simulink model "cmd_model"  (R2015a)
settings: configuration reference "config_cosim" (kept outside this file)
libraries: Sys_CMD x1
settings Model: Creator=ericli  LastModifiedBy=ericli
settings ConfigSetRef: SourceLocation=Base Workspace

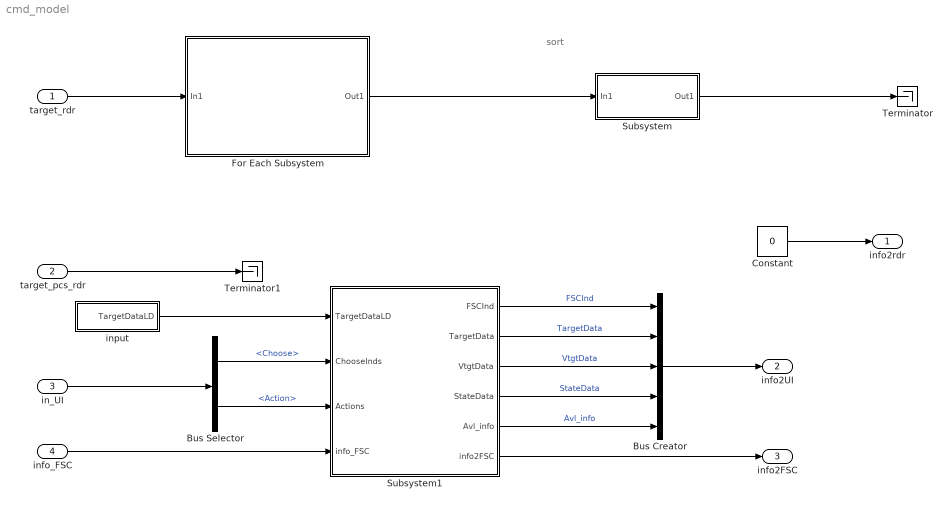
== system cmd_model ==
  note: sort
  target_rdr : Inport  OutDataTypeStr=Bus: BusObject_tgt_rdr2CC  PortDimensions=48  BusOutputAsStruct=on
  target_pcs_rdr : Inport  Port=2  OutDataTypeStr=Bus: BusObject_msg_pcs_rdr2CC  BusOutputAsStruct=on
  in_UI : Inport  Port=3  OutDataTypeStr=Bus: BusObject_input_UI  BusOutputAsStruct=on
  info_FSC : Inport  Port=4  OutDataTypeStr=Bus: BusObject_info_FSC2CC
  Bus Creator : BusCreator  Inputs=5  OutDataTypeStr=Bus: BusObject_info_CC2UI
      settings: InheritFromInputs=off
  Bus Selector : BusSelector  OutputSignals=Choose,Action
  Constant : Constant  Value=0  OutDataTypeStr=Bus:BusObject_info_CC2rdr  LockScale=on
  For Each Subsystem : Subsystem  TreatAsAtomicUnit=on
  Subsystem : Subsystem
  Subsystem1 : Subsystem
  Terminator : Terminator
  Terminator1 : Terminator
  input : Subsystem
  info2rdr : Outport  OutDataTypeStr=Bus: BusObject_info_CC2rdr  BusOutputAsStruct=on
  info2UI : Outport  Port=2  OutDataTypeStr=Bus: BusObject_info_CC2UI
  info2FSC : Outport  Port=3  OutDataTypeStr=Bus: BusObject_info_CC2FSC
  wires:
  target_rdr/1 -> For Each Subsystem/1(In1)
  For Each Subsystem/1(Out1) -> Subsystem/1(In1)
  Subsystem/1(Out1) -> Terminator/1
  Bus Creator/1 -> info2UI/1
  in_UI/1 -> Bus Selector/1
  Bus Selector/1 -> Subsystem1/2(ChooseInds)  "<Choose>"
  Bus Selector/2 -> Subsystem1/3(Actions)  "<Action>"
  info_FSC/1 -> Subsystem1/4(info_FSC)
  Subsystem1/6(info2FSC) -> info2FSC/1
  Constant/1 -> info2rdr/1
  Subsystem1/5(Avl_info) -> Bus Creator/5  "Avl_info"
  Subsystem1/4(StateData) -> Bus Creator/4  "StateData"
  Subsystem1/2(TargetData) -> Bus Creator/2  "TargetData"
  Subsystem1/1(FSCInd) -> Bus Creator/1  "FSCInd"
  input/1(TargetDataLD) -> Subsystem1/1(TargetDataLD)
  target_pcs_rdr/1 -> Terminator1/1
  Subsystem1/3(VtgtData) -> Bus Creator/3  "VtgtData"

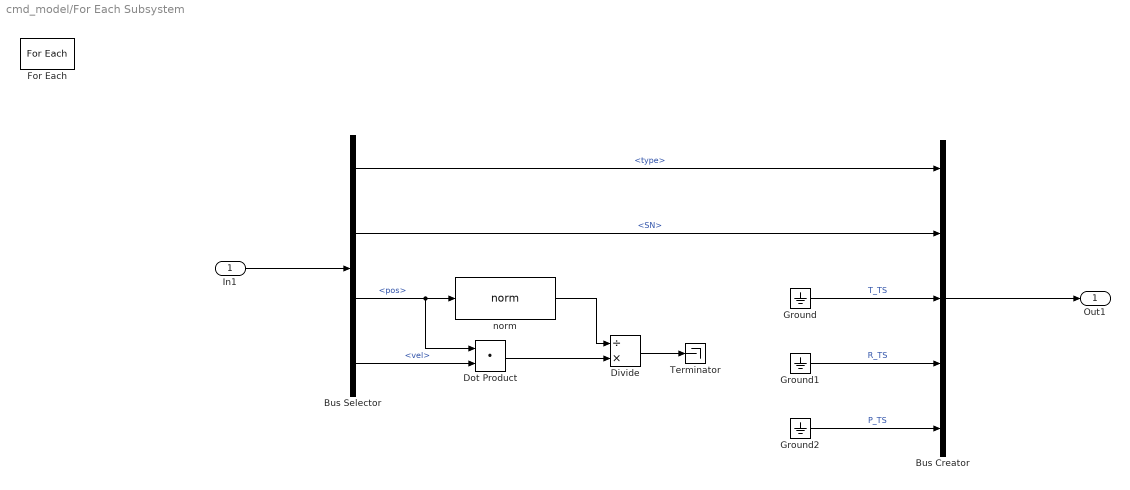
== system cmd_model/For Each Subsystem ==
  In1 : Inport  Partition=on  PartitionDimension=1  PartitionWidth=1
  Bus Creator : BusCreator  Inputs=5  OutDataTypeStr=Bus: bus_cmp_tgt  NonVirtualBus=on
      settings: InheritFromInputs=off
  Bus Selector : BusSelector  OutputSignals=type,SN,pos,vel
  Divide : Product  Inputs=/*
  Dot Product : DotProduct  InputSameDT=on  OutDataTypeStr=Inherit: Inherit via internal rule
  For Each : ForEach  DisableCoverage=on  IndexMode=One-based
  Ground : Ground
  Ground1 : Ground
  Ground2 : Ground
  Terminator : Terminator
  norm : Sys_CMD/norm
  Out1 : Outport  OutDataTypeStr=Bus: bus_cmp_tgt  ConcatenationDimension=1
  wires:
  In1/1 -> Bus Selector/1
  Bus Selector/3 -> norm/1, Dot Product/1  "<pos>"
  Bus Selector/4 -> Dot Product/2  "<vel>"
  norm/1 -> Divide/1
  Dot Product/1 -> Divide/2
  Divide/1 -> Terminator/1
  Bus Creator/1 -> Out1/1
  Bus Selector/1 -> Bus Creator/1  "<type>"
  Bus Selector/2 -> Bus Creator/2  "<SN>"
  Ground/1 -> Bus Creator/3  "T_TS"
  Ground1/1 -> Bus Creator/4  "R_TS"
  Ground2/1 -> Bus Creator/5  "P_TS"

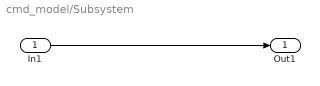
== system cmd_model/Subsystem ==
  In1 : Inport
  Out1 : Outport
  wires:
  In1/1 -> Out1/1

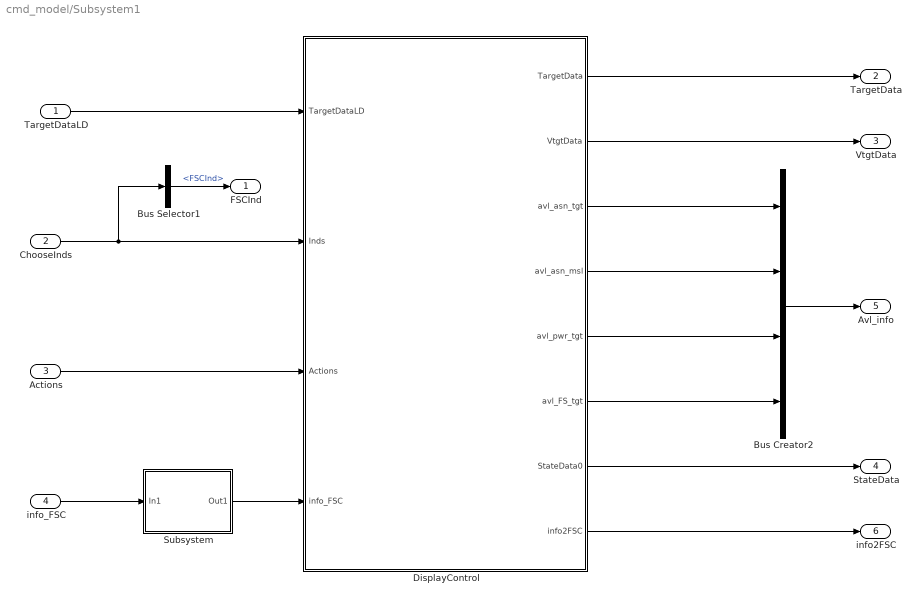
== system cmd_model/Subsystem1 ==
  TargetDataLD : Inport
  ChooseInds : Inport  Port=2  OutDataTypeStr=Bus:ChooseBusObject
  Actions : Inport  Port=3  OutDataTypeStr=Bus: ActionBusObject
  info_FSC : Inport  Port=4  OutDataTypeStr=Bus:BusObject_info_FSC2CC
  Bus Creator2 : BusCreator  OutDataTypeStr=Bus:AvlBusObject
  Bus Selector1 : BusSelector  OutputSignals=FSCInd
  DisplayControl : Stateflow chart  TreatAsAtomicUnit=on
  Subsystem : Subsystem
  FSCInd : Outport
  TargetData : Outport  Port=2
  VtgtData : Outport  Port=3
  StateData : Outport  Port=4  OutDataTypeStr=Bus:StateBusObject
  Avl_info : Outport  Port=5  OutDataTypeStr=Bus:AvlBusObject
  info2FSC : Outport  Port=6  OutDataTypeStr=Bus: BusObject_info_CC2FSC
  wires:
  DisplayControl/3(avl_asn_tgt) -> Bus Creator2/1
  DisplayControl/8(info2FSC) -> info2FSC/1
  DisplayControl/1(TargetData) -> TargetData/1
  Bus Creator2/1 -> Avl_info/1
  TargetDataLD/1 -> DisplayControl/1(TargetDataLD)
  DisplayControl/5(avl_pwr_tgt) -> Bus Creator2/3
  DisplayControl/7(StateData0) -> StateData/1
  DisplayControl/4(avl_asn_msl) -> Bus Creator2/2
  Bus Selector1/1 -> FSCInd/1  "<FSCInd>"
  ChooseInds/1 -> DisplayControl/2(Inds), Bus Selector1/1
  DisplayControl/6(avl_FS_tgt) -> Bus Creator2/4
  Actions/1 -> DisplayControl/3(Actions)
  DisplayControl/2(VtgtData) -> VtgtData/1
  info_FSC/1 -> Subsystem/1(In1)
  Subsystem/1(Out1) -> DisplayControl/4(info_FSC)

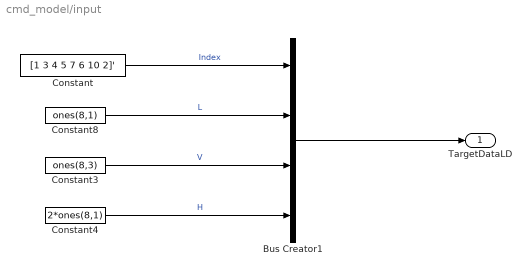
== system cmd_model/input ==
  Bus Creator1 : BusCreator  OutDataTypeStr=Bus: TgtDataLDBusObject  NonVirtualBus=on
  Constant : Constant  Value=[1 3 4 5 7 6 10 2]'  OutDataTypeStr=double
  Constant3 : Constant  Value=ones(8,3)  OutDataTypeStr=double
  Constant4 : Constant  Value=2*ones(8,1)  OutDataTypeStr=double
  Constant8 : Constant  Value=ones(8,1)  OutDataTypeStr=double
  TargetDataLD : Outport  OutDataTypeStr=Bus: TgtDataLDBusObject
  wires:
  Constant8/1 -> Bus Creator1/2  "L"
  Constant4/1 -> Bus Creator1/4  "H"
  Constant/1 -> Bus Creator1/1  "Index"
  Constant3/1 -> Bus Creator1/3  "V"
  Bus Creator1/1 -> TargetDataLD/1

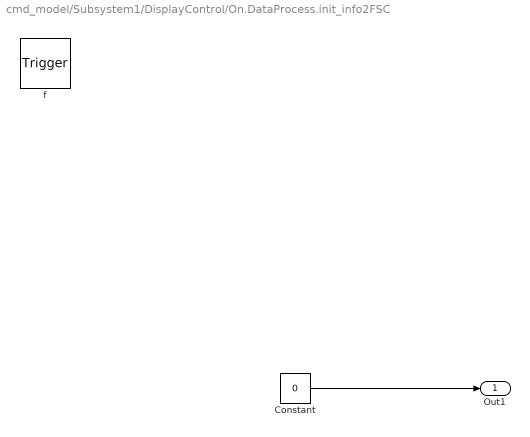
== system cmd_model/Subsystem1/DisplayControl/On.DataProcess.init_info2FSC ==
  f : TriggerPort  TriggerType=function-call
      settings: CopyFcn=Stateflow.SLINSF.SimulinkMan.removeBlockPreDeleteFcn  PreDeleteFcn=Stateflow.SLINSF.SimulinkMan.unsafePredeleteFcn
  Constant : Constant  Value=0  OutDataTypeStr=Bus: BusObject_info_CC2FSC
  Out1 : Outport  OutDataTypeStr=Bus: BusObject_info_CC2FSC
  wires:
  Constant/1 -> Out1/1

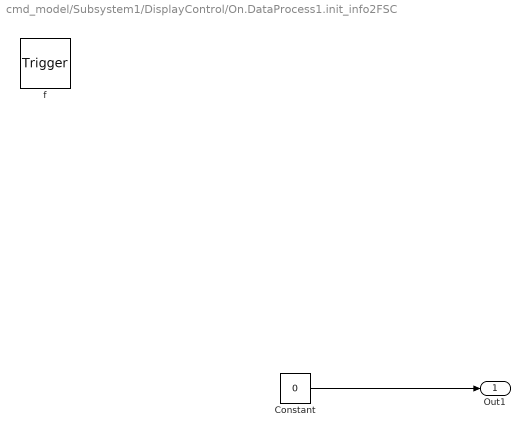
== system cmd_model/Subsystem1/DisplayControl/On.DataProcess1.init_info2FSC ==
  f : TriggerPort  TriggerType=function-call
      settings: CopyFcn=Stateflow.SLINSF.SimulinkMan.removeBlockPreDeleteFcn  PreDeleteFcn=Stateflow.SLINSF.SimulinkMan.unsafePredeleteFcn
  Constant : Constant  Value=0  OutDataTypeStr=Bus: BusObject_info_CC2FSC
  Out1 : Outport  OutDataTypeStr=Bus: BusObject_info_CC2FSC
  wires:
  Constant/1 -> Out1/1

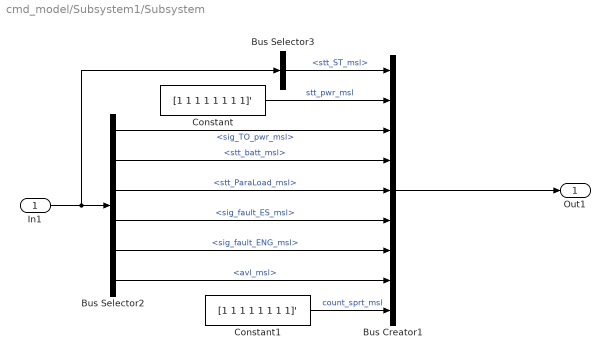
== system cmd_model/Subsystem1/Subsystem ==
  In1 : Inport
  Bus Creator1 : BusCreator  Inputs=9  OutDataTypeStr=Bus:BusObject_info_FSC2CC
  Bus Selector2 : BusSelector  OutputSignals=sig_TO_pwr_msl,stt_batt_msl,stt_ParaLoad_msl,sig_fault_ES_msl,sig_fault_ENG_msl,avl_msl
  Bus Selector3 : BusSelector  OutputSignals=stt_ST_msl
  Constant : Constant  Value=[1 1 1 1 1 1 1 1]'  OutDataTypeStr=boolean
  Constant1 : Constant  Value=[1 1 1 1 1 1 1 1]'  OutDataTypeStr=double
  Out1 : Outport
  wires:
  Bus Selector2/1 -> Bus Creator1/3  "<sig_TO_pwr_msl>"
  Bus Selector2/2 -> Bus Creator1/4  "<stt_batt_msl>"
  Bus Creator1/1 -> Out1/1
  Constant1/1 -> Bus Creator1/9  "count_sprt_msl"
  Bus Selector2/4 -> Bus Creator1/6  "<sig_fault_ES_msl>"
  Bus Selector2/5 -> Bus Creator1/7  "<sig_fault_ENG_msl>"
  Constant/1 -> Bus Creator1/2  "stt_pwr_msl"
  Bus Selector2/3 -> Bus Creator1/5  "<stt_ParaLoad_msl>"
  Bus Selector3/1 -> Bus Creator1/1  "<stt_ST_msl>"
  Bus Selector2/6 -> Bus Creator1/8  "<avl_msl>"
  In1/1 -> Bus Selector3/1, Bus Selector2/1

== stateflow chart cmd_model/Subsystem1/DisplayControl ==
  settings: executeAtInitialization=1
  state Init
    entry:
    TargetData(:,1) = TargetDataLD.L;
    TargetData(:,3) = TargetDataLD.H;
    VtgtData = TargetDataLD.V;
    TargetData(:,7) = TargetDataLD.Index;
    StateData = zeros(8,3);
    StateInf = 0;
    avl_asn_msl = ones(8,1);
    avl_FS_tgt = zeros(8,1);
    avl_pwr_tgt = zeros(8,1);
  state On
    state TargetPower [parallel]
      % 根据选择的目标更新加电和断电信息
      settings: executionOrder=4
      TargetPower -> (junction 337)
      (junction 337) -> (junction 441) [order 1] : [Actions.TgtAsn]
      (junction 337) -> (junction 339) [order 2]
      (junction 441) -> (junction 443) : {avl_pwr_tgt(Inds.TgtAsnInd) = 1;}
      (junction 443) -> (junction 339)
      (junction 339) -> (junction 687)
      (junction 687) -> (junction 685) [order 1] : [Actions.TgtAsnCcl]
      (junction 687) -> (junction 684) [order 2]
      (junction 685) -> (junction 691) : {avl_pwr_tgt(Inds.TgtAsnInd) = 0;}
      (junction 691) -> (junction 684)
    state DataProcess [parallel] [commented out]
      entry:
      Para_FS0.pos_tgt = [0;0;0];
      Para_FS0.vel_tgt = [0;0;0];
      info2FSC.Para_FS(1:8) = Para_FS0;
      info2FSC.ins_pwr_on =  false(8,1);
      info2FSC.ins_pwr_of = [false;false;false;false;false;false;false;false];
      info2FSC.ins_FS = [false;false;false;false;false;false;false;false];
      state FS [parallel] [commented out]
        (default) -> (junction 914) [commented out]
        On.DataProcess.FS -> (junction 914) [commented out]
        (junction 914) -> (junction 905) [commented out] : [Actions.FS]
        (junction 914) -> (junction 902) [commented out]
        (junction 905) -> (junction 910) [commented out] : {info2FSC.ins_pwr_on = [false;false;false;false;false;false;false;false];
            | info2FSC.ins_pwr_of = [false;false;false;false;false;false;false;false];
            | info2FSC.ins_FS = [false;false;false;false;false;false;false;false];}
        (junction 910) -> (junction 902) [commented out]
        (junction 902) -> (junction 1221) [commented out] : {i = 1;}
        (junction 913) -> (junction 922) [commented out] : [Inds.TgtFsInd(i,1)]
        (junction 1221) -> (junction 913) [commented out] : [i  < 8]
        (junction 913) -> (junction 907) [commented out]
        (junction 922) -> (junction 1201) [commented out] : {ddInd1 = TargetData(i,5);
            | info2FSC.ins_FS(ddInd1) = true;}
        (junction 1201) -> (junction 907) [commented out]
        (junction 907) -> (junction 919) [commented out]
        (junction 916) -> (junction 1221) [commented out] : {i = i + 1;}
        (junction 1221) -> (junction 1222) [commented out]
        (junction 919) -> (junction 918) [commented out] : [Inds.TgtFsInd(i,2)]
        (junction 918) -> (junction 1203) [commented out] : {ddInd1 = TargetData(i,6);
            | info2FSC.ins_FS(ddInd1) = true;}
        (junction 919) -> (junction 916) [commented out]
        (junction 1203) -> (junction 916) [commented out]
      state DataUpdateWithFSCInfo [parallel] [commented out]
        (default) -> (junction 981) [commented out] : {avl_asn_msl =double(avl_asn_msl&info_FSC.avl_msl);}
        On.DataProcess.DataUpdateWithFSCInfo -> (junction 981) [commented out]
        (junction 981) -> (junction 980) [commented out] : {m = 0;
            | n = 0;
            | j = 1;}
        (junction 979) -> (junction 968) [commented out] : % 导弹出现故障
            | [~info_FSC.avl_msl(j)]
        (junction 980) -> (junction 979) [commented out] : [j  < 8]
        (junction 979) -> (junction 972) [commented out]
        (junction 968) -> (junction 994) [commented out] : {StateData(j,1:3) =2;}
        (junction 972) -> (junction 984) [commented out] : %虽然有加电命令，但是加电状态为未加电
            | [info2FSC.ins_pwr_on(j)==1 && info_FSC.stt_pwr_msl(j) ==0]
        (junction 977) -> (junction 980) [commented out] : {j = j + 1;}
        (junction 980) -> (junction 1177) [commented out]
        (junction 972) -> (junction 973) [commented out]
        (junction 984) -> (junction 988) [commented out] : {StateData(j,2) = 0;
            | m = m+1;}
        (junction 973) -> (junction 966) [commented out] : %虽然有发射命令，但是离架计时为0，说明没有发生
            | [info2FSC.ins_FS(j)==1 && info_FSC.count_sprt_msl(j)<=0]
        (junction 973) -> (junction 977) [commented out]
        (junction 966) -> (junction 991) [commented out] : {StateData(j,3) = 0;
            | n = n+1;}
        (junction 991) -> (junction 977) [commented out]
        (junction 988) -> (junction 991) [commented out]
        (junction 994) -> (junction 988) [commented out]
        (junction 1177) -> (junction 1173) [commented out] : [Actions.PwrOn||Actions.PwrOff||Actions.FS]
        (junction 1177) -> (junction 1174) [commented out]
        (junction 1173) -> (junction 1178) [commented out] : {StateInf = 0;}
        (junction 1178) -> (junction 1174) [commented out]
        (junction 1174) -> (junction 999) [commented out]
        (junction 999) -> (junction 1001) [commented out] : [sum(info2FSC.ins_pwr_on)>0&&m == sum(info2FSC.ins_pwr_on)] % 说明本次没有加电成功的DD
        (junction 999) -> (junction 1005) [commented out]
        (junction 1001) -> (junction 1003) [commented out] : {StateInf = 712;}
        (junction 1003) -> (junction 1005) [commented out]
        (junction 1005) -> (junction 1009) [commented out]
        (junction 1009) -> (junction 1011) [commented out] : [sum(info2FSC.ins_FS)>0&&n == sum(info2FSC.ins_FS)] % 说明本次没有发射成功的DD
        (junction 1009) -> (junction 1008) [commented out]
        (junction 1011) -> (junction 1012) [commented out] : {StateInf = 110;}
        (junction 1012) -> (junction 1008) [commented out]
        (junction 1008) -> (junction 1021) [commented out] : {StateData0.StateData = StateData;
            | StateData0.StateInf = StateInf;
            | j = 1;}
        (junction 1024) -> (junction 1040) [commented out] : [avl_FS_tgt(j) == 1]
        (junction 1040) -> (junction 1086) [commented out] : % 选了j个目标的第1颗dd
            | [Inds.TgtPwrInd(j,1)]
        (junction 1021) -> (junction 1024) [commented out] : [j<8]
        (junction 1024) -> (junction 1208) [commented out]
        (junction 1040) -> (junction 1098) [commented out] : {DD1 = 0;
            | DD10 = 0; }
        (junction 1086) -> (junction 1088) [commented out] : %j个目标的第一颗dd编号
            | {DD1 = TargetData(j,5);}
        (junction 1088) -> (junction 1098) [commented out]
        (junction 1098) -> (junction 1106) [commented out]
        (junction 1106) -> (junction 1104) [commented out] : [DD1>0]
        (junction 1104) -> (junction 1105) [commented out] : %这颗dd的状态为0
            | [info_FSC.stt_pwr_msl(DD1)==0]
        (junction 1106) -> (junction 1110) [commented out]
        (junction 1104) -> (junction 1141) [commented out] : {DD10 = 1;}
        (junction 1105) -> (junction 1112) [commented out] : %选中了dd1且dd1状态为0
            | {DD10 = 0;}
        (junction 1141) -> (junction 1110) [commented out]
        (junction 1112) -> (junction 1141) [commented out]
        (junction 1110) -> (junction 1092) [commented out]
        (junction 1208) -> (junction 1021) [commented out] : {j = j+1;}
        (junction 1021) -> (junction 1034) [commented out]
        (junction 1092) -> (junction 1096) [commented out] : [Inds.TgtPwrInd(j,2)]
        (junction 1092) -> (junction 1101) [commented out] : {DD2 = 0;
            | DD20= 0;}
        (junction 1096) -> (junction 1094) [commented out] : {DD2 = TargetData(j,6);}
        (junction 1094) -> (junction 1101) [commented out]
        (junction 1101) -> (junction 1125) [commented out]
        (junction 1125) -> (junction 1126) [commented out] : [DD2>0]
        (junction 1126) -> (junction 1127) [commented out] : [info_FSC.stt_pwr_msl(DD2)==0]
        (junction 1125) -> (junction 1118) [commented out]
        (junction 1126) -> (junction 1143) [commented out] : {DD20 = 1;}
        (junction 1127) -> (junction 1122) [commented out] : {DD20 = 0;}
        (junction 1143) -> (junction 1118) [commented out]
        (junction 1122) -> (junction 1143) [commented out]
        (junction 1118) -> (junction 1036) [commented out]
        (junction 1036) -> (junction 1048) [commented out] : % 两颗dd均被选，但是两颗dd的状态均为0
            | % 或者一颗dd选中了，其状态为0，而另一颗dd未选
            | [DD10==0&&DD20==0]
        (junction 1036) -> (junction 1138) [commented out]
        (junction 1048) -> (junction 1137) [commented out] : {avl_FS_tgt(j) = 0;}
        (junction 1138) -> (junction 1208) [commented out]
        (junction 1137) -> (junction 1138) [commented out]
      state PwrOff [parallel] [commented out]
        (default) -> (junction 889) [commented out]
        On.DataProcess.PwrOff -> (junction 889) [commented out]
        (junction 889) -> (junction 880) [commented out] : [Actions.PwrOff]
        (junction 889) -> (junction 877) [commented out]
        (junction 880) -> (junction 885) [commented out] : {info2FSC.ins_pwr_on = [false;false;false;false;false;false;false;false];
            | info2FSC.ins_pwr_of = [false;false;false;false;false;false;false;false];
            | info2FSC.ins_FS = [false;false;false;false;false;false;false;false];}
        (junction 885) -> (junction 877) [commented out]
        (junction 877) -> (junction 1217) [commented out] : {i = 1;}
        (junction 888) -> (junction 897) [commented out] : [Inds.TgtPwrInd(i,1)]
        (junction 1217) -> (junction 888) [commented out] : [i  < 8]
        (junction 888) -> (junction 882) [commented out]
        (junction 897) -> (junction 1197) [commented out] : {ddInd1 = TargetData(i,5);
            | info2FSC.ins_pwr_of(ddInd1) = true;}
        (junction 1197) -> (junction 882) [commented out]
        (junction 891) -> (junction 1217) [commented out] : {i = i + 1;}
        (junction 1217) -> (junction 1219) [commented out]
        (junction 882) -> (junction 894) [commented out]
        (junction 894) -> (junction 893) [commented out] : [Inds.TgtPwrInd(i,2)]
        (junction 894) -> (junction 891) [commented out]
        (junction 893) -> (junction 1199) [commented out] : {ddInd1 = TargetData(i,6);
            | info2FSC.ins_pwr_of(ddInd1) = true;}
        (junction 1199) -> (junction 891) [commented out]
      state PwrOn [parallel] [commented out]
        (default) -> (junction 863) [commented out]
        On.DataProcess.PwrOn -> (junction 863) [commented out]
        (junction 863) -> (junction 852) [commented out] : [Actions.PwrOn]
        (junction 863) -> (junction 853) [commented out]
        (junction 852) -> (junction 851) [commented out] : {info2FSC.ins_pwr_on = [false;false;false;false;false;false;false;false];
            | info2FSC.ins_pwr_of = [false;false;false;false;false;false;false;false];
            | info2FSC.ins_FS = [false;false;false;false;false;false;false;false];}
        (junction 851) -> (junction 853) [commented out]
        (junction 862) -> (junction 864) [commented out] : [Inds.TgtPwrInd(i,1)]
        (junction 1214) -> (junction 862) [commented out] : [i  < 8]
        (junction 853) -> (junction 1214) [commented out] : {i = 1;}
        (junction 862) -> (junction 857) [commented out]
        (junction 864) -> (junction 1193) [commented out] : {ddInd1 = TargetData(i,5);
            | info2FSC.ins_pwr_on(ddInd1) = true;}
        (junction 1193) -> (junction 857) [commented out]
        (junction 857) -> (junction 870) [commented out]
        (junction 869) -> (junction 1214) [commented out] : {i = i + 1;}
        (junction 1214) -> (junction 1212) [commented out]
        (junction 870) -> (junction 871) [commented out] : [Inds.TgtPwrInd(i,2)]
        (junction 870) -> (junction 869) [commented out]
        (junction 871) -> (junction 1195) [commented out] : {ddInd1 = TargetData(i,6);
            | info2FSC.ins_pwr_on(ddInd1) = true;}
        (junction 1195) -> (junction 869) [commented out]
      state Out1 = init_info2FSC [function] [commented out]
    state TargetDataProcess [parallel]
      settings: executionOrder=1
      state Time
      (default) -> Time : {TargetData(:,1) = TargetDataLD.L;
          | TargetData(:,3) = TargetDataLD.H;
          | VtgtData = TargetDataLD.V;
          | TargetData(:,7) = TargetDataLD.Index;}
      Time -> TargetDataProcess : [after(1,sec)]
    state DataUpdate [parallel]
      % 根据状态更新状态信息以及表格中要显示的数据
      en:StateData = zeros(8,3);
      settings: executionOrder=2
      state FS [parallel]
        settings: executionOrder=3
        (junction 611) -> (junction 604) [order 1] : [i  < 8]
        (junction 604) -> (junction 607)
        On.DataUpdate.FS -> (junction 605)
        (junction 605) -> (junction 606) [order 1] : [Actions.FS]
        (junction 605) -> (junction 812) [order 2]
        (junction 606) -> (junction 611) : {i = 1;}
        (junction 607) -> (junction 608) [order 1] : [Inds.TgtFsInd(i,1)>0]
        (junction 607) -> (junction 609) [order 2]
        (junction 608) -> (junction 610) : {ddInd = TargetData(i,5);
            | StateData(ddInd,3) = 1;}
        (junction 610) -> (junction 609)
        (junction 609) -> (junction 612)
        (junction 617) -> (junction 611) : {i = i + 1;}
        (junction 611) -> (junction 616) [order 2]
        (junction 612) -> (junction 613) [order 1] : [Inds.TgtFsInd(i,2)>0]
        (junction 612) -> (junction 614) [order 2]
        (junction 613) -> (junction 615) : {ddInd = TargetData(i,6);
            | StateData(ddInd,3) = 1;}
        (junction 615) -> (junction 614)
        (junction 812) -> (junction 616)
        (junction 614) -> (junction 617)
      state Assign [parallel]
        settings: executionOrder=1
        Assign -> (junction 412)
        (junction 412) -> (junction 416) [order 1] : [Inds.TgtAsnInd>0&&Actions.TgtAsn]
        (junction 412) -> (junction 415) [order 2]
        (junction 416) -> (junction 410) : {TargetData(Inds.TgtAsnInd,5) = ((Inds.FSCInd-1)*2+1)*Inds.MslInd(1);
            |  TargetData(Inds.TgtAsnInd,6) = ((Inds.FSCInd-1)*2+2)*Inds.MslInd(2);}
        (junction 410) -> (junction 447) [order 1] : [Inds.MslInd(1)]
        (junction 410) -> (junction 815) [order 2]
        (junction 447) -> (junction 814) : {StateData((Inds.FSCInd-1)*2+1,1) = 1;}
        (junction 814) -> (junction 815)
        (junction 815) -> (junction 449)
        (junction 449) -> (junction 452) [order 1] : [Inds.MslInd(2)]
        (junction 449) -> (junction 454) [order 2]
        (junction 452) -> (junction 818) : {StateData((Inds.FSCInd-1)*2+2,1) = 1;}
        (junction 454) -> (junction 415)
        (junction 818) -> (junction 454)
        (junction 415) -> (junction 662)
        (junction 662) -> (junction 664) [order 1] : [Inds.TgtAsnInd>0&&Actions.TgtAsnCcl]
        (junction 664) -> (junction 679) [order 1] : [Inds.FSCInd]
        (junction 662) -> (junction 665) [order 2]
        (junction 664) -> (junction 676) [order 2]
        (junction 679) -> (junction 820) : {TargetData(Inds.TgtAsnInd,5) = 0;
            |  TargetData(Inds.TgtAsnInd,6) = 0;
            | StateData((Inds.FSCInd-1)*2+1,1) = 0;
            | StateData((Inds.FSCInd-1)*2+2,1) = 0;}
        (junction 676) -> (junction 665)
        (junction 820) -> (junction 676)
      state Pwr [parallel]
        settings: executionOrder=2
        (junction 532) -> (junction 530) [order 1] : [i  < 8]
        (junction 530) -> (junction 544)
        (junction 544) -> (junction 543) [order 1] : [Inds.TgtPwrInd(i,1)>0]
        (junction 544) -> (junction 545) [order 2]
        (junction 543) -> (junction 542) : {ddInd = TargetData(i,5);
            | StateData(ddInd,2) = 1;}
        (junction 542) -> (junction 545)
        (junction 545) -> (junction 559)
        Pwr -> (junction 484)
        (junction 484) -> (junction 531) [order 1] : [Actions.PwrOn]
        (junction 559) -> (junction 553) [order 1] : [Inds.TgtPwrInd(i,2)>0]
        (junction 484) -> (junction 809) [order 2]
        (junction 531) -> (junction 532) : {i = 1;}
        (junction 559) -> (junction 554) [order 2]
        (junction 553) -> (junction 552) : {ddInd = TargetData(i,6);
            | StateData(ddInd,2) = 1;}
        (junction 552) -> (junction 554)
        (junction 554) -> (junction 533)
        (junction 735) -> (junction 718) [order 1] : [i  < 8]
        (junction 718) -> (junction 728)
        (junction 533) -> (junction 532) : {i = i + 1;}
        (junction 532) -> (junction 534) [order 2]
        (junction 728) -> (junction 727) [order 1] : [Inds.TgtPwrInd(i,1)>0]
        (junction 728) -> (junction 719) [order 2]
        (junction 727) -> (junction 725) : {ddInd = TargetData(i,5);
            | StateData(ddInd,2) = 0;}
        (junction 534) -> (junction 716) [order 1] : [Actions.PwrOff]
        (junction 809) -> (junction 534)
        (junction 725) -> (junction 719)
        (junction 534) -> (junction 808) [order 2]
        (junction 716) -> (junction 735) : {i = 1;}
        (junction 719) -> (junction 723)
        (junction 723) -> (junction 733) [order 1] : [Inds.TgtPwrInd(i,2)>0]
        (junction 723) -> (junction 724) [order 2]
        (junction 733) -> (junction 721) : {ddInd = TargetData(i,6);
            | StateData(ddInd,2) = 0;}
        (junction 721) -> (junction 724)
        (junction 724) -> (junction 732)
        (junction 732) -> (junction 735) : {i = i + 1;}
        (junction 735) -> (junction 744) [order 2]
        (junction 808) -> (junction 744)
    state TargetAssign [parallel]
      % 根据选择的目标、FSC和DD更新可分配的目标、FSC和DD数据
      en:avl_asn_tgt = ones(8,1);
      settings: executionOrder=3
      (junction 328) -> (junction 330) [order 1] : [Actions.TgtAsn]
      TargetAssign -> (junction 328)
      (junction 330) -> (junction 421) : {avl_asn_tgt(Inds.TgtAsnInd) = 0;}
      (junction 328) -> (junction 329) [order 2]
      (junction 421) -> (junction 423) [order 1] : [Inds.MslInd(1)>0]
      (junction 421) -> (junction 824) [order 2]
      (junction 423) -> (junction 826) : {avl_asn_msl((Inds.FSCInd-1)*2+1) = 0;}
      (junction 826) -> (junction 824)
      (junction 824) -> (junction 430)
      (junction 430) -> (junction 436) [order 1] : [Inds.MslInd(2)>0]
      (junction 430) -> (junction 434) [order 2]
      (junction 436) -> (junction 822) : {avl_asn_msl((Inds.FSCInd-1)*2+2) = 0;}
      (junction 434) -> (junction 329)
      (junction 822) -> (junction 434)
      (junction 329) -> (junction 637)
      (junction 637) -> (junction 655) [order 1] : [Actions.TgtAsnCcl]
      (junction 655) -> (junction 641) : {avl_asn_tgt(Inds.TgtAsnInd) = 1;}
      (junction 637) -> (junction 639) [order 2]
      (junction 641) -> (junction 647) [order 1] : [Inds.MslInd(1)>0]
      (junction 641) -> (junction 831) [order 2]
      (junction 647) -> (junction 830) : {avl_asn_msl((Inds.FSCInd-1)*2+1) = 1;}
      (junction 830) -> (junction 831)
      (junction 831) -> (junction 646)
      (junction 646) -> (junction 648) [order 1] : [Inds.MslInd(2)>0]
      (junction 648) -> (junction 828) : {avl_asn_msl((Inds.FSCInd-1)*2+2) = 1;}
      (junction 646) -> (junction 643) [order 2]
      (junction 643) -> (junction 639)
      (junction 828) -> (junction 643)
    state FS [parallel]
      % 根据选择的目标更新DD发射信息
      settings: executionOrder=5
      On.FS -> (junction 587)
      (junction 587) -> (junction 585) [order 1] : [Actions.PwrOn]
      (junction 587) -> (junction 693) [order 2]
      (junction 585) -> (junction 577) : {i = 1;}
      (junction 577) -> (junction 693) [order 2]
      (junction 577) -> (junction 590) [order 1] : [i  < 8]
      (junction 590) -> (junction 597) [order 1] : [Inds.TgtPwrInd(i,1)||Inds.TgtPwrInd(i,2)]
      (junction 571) -> (junction 577) : {i = i + 1;}
      (junction 693) -> (junction 707)
      (junction 590) -> (junction 571) [order 2]
      (junction 597) -> (junction 1185) : {avl_FS_tgt(i) = 1;}
      (junction 1185) -> (junction 571)
      (junction 707) -> (junction 700) [order 1] : [Actions.PwrOff]
      (junction 707) -> (junction 708) [order 2]
      (junction 700) -> (junction 704) : {i = 1;}
      (junction 704) -> (junction 708) [order 2]
      (junction 704) -> (junction 771) [order 1] : [i  < 8]
      (junction 771) -> (junction 770) [order 1] : [Inds.TgtPwrInd(i,1)]
      (junction 796) -> (junction 704) : {i = i + 1;}
      (junction 771) -> (junction 747) [order 2]
      (junction 770) -> (junction 777) : %该目标的配置的另一个DD
          | {ddInd = TargetData(i,6);}
      (junction 777) -> (junction 798) [order 1] : [ddInd==0||(ddInd~=0&&StateData(ddInd,2) == 0)]
      (junction 777) -> (junction 778) [order 2]
      (junction 798) -> (junction 1187) : {avl_FS_tgt(i) = 0;}
      (junction 778) -> (junction 747)
      (junction 1187) -> (junction 778)
      (junction 747) -> (junction 754)
      (junction 754) -> (junction 769) [order 1] : [Inds.TgtPwrInd(i,2)]
      (junction 754) -> (junction 796) [order 2]
      (junction 769) -> (junction 788) : {ddInd = TargetData(i,5);}
      (junction 788) -> (junction 804) [order 1] : [ddInd==0||(ddInd~=0&&StateData(ddInd,1) == 0)]
      (junction 788) -> (junction 1189) [order 2]
      (junction 804) -> (junction 806) : {avl_FS_tgt(i) = 0;}
      (junction 1189) -> (junction 796)
      (junction 806) -> (junction 1189)
    state DataProcess1 [parallel]
      en:
      info2FSC = struct_info_CC2FSC;
      settings: executionOrder=6
      state FS [parallel]
        settings: executionOrder=3
        (default) -> (junction 1390)
        On.DataProcess1.FS -> (junction 1390)
        (junction 1390) -> (junction 1391) [order 1] : [Actions.FS]
        (junction 1391) -> (junction 1393) : {info2FSC.ins_pwr_on = [false;false;false;false;false;false;false;false];
            | info2FSC.ins_pwr_of = [false;false;false;false;false;false;false;false];
            | info2FSC.ins_FS = [false;false;false;false;false;false;false;false];}
        (junction 1390) -> (junction 1392) [order 2]
        (junction 1393) -> (junction 1392)
        (junction 1392) -> (junction 1398) : {i = 1;}
        (junction 1394) -> (junction 1395) [order 1] : [Inds.TgtFsInd(i,1)]
        (junction 1398) -> (junction 1394) [order 1] : [i  < 8]
        (junction 1394) -> (junction 1396) [order 2]
        (junction 1395) -> (junction 1397) : {ddInd1 = TargetData(i,5);
            | info2FSC.ins_FS(ddInd1) = true;}
        (junction 1397) -> (junction 1396)
        (junction 1396) -> (junction 1399)
        (junction 1403) -> (junction 1398) : {i = i + 1;}
        (junction 1398) -> (junction 1402) [order 2]
        (junction 1399) -> (junction 1400) [order 1] : [Inds.TgtFsInd(i,2)]
        (junction 1400) -> (junction 1401) : {ddInd1 = TargetData(i,6);
            | info2FSC.ins_FS(ddInd1) = true;}
        (junction 1399) -> (junction 1403) [order 2]
        (junction 1401) -> (junction 1403)
      state DataUpdateWithFSCInfo [parallel]
        settings: executionOrder=4
        (default) -> (junction 1268) : {avl_asn_msl =double(avl_asn_msl&info_FSC.avl_msl);}
        On.DataProcess1.DataUpdateWithFSCInfo -> (junction 1268)
        (junction 1268) -> (junction 1271) : {m = 0;
            | n = 0;
            | j = 1;}
        (junction 1269) -> (junction 1270) [order 1] : % 导弹出现故障
            | [~info_FSC.avl_msl(j)]
        (junction 1271) -> (junction 1269) [order 1] : [j  < 8]
        (junction 1269) -> (junction 1272) [order 2]
        (junction 1270) -> (junction 1279) : {StateData(j,1:3) =2;}
        (junction 1272) -> (junction 1273) [order 1] : %虽然有加电命令，但是加电状态为未加电
            | [info2FSC.ins_pwr_on(j)==1 && info_FSC.stt_pwr_msl(j) ==0]
        (junction 1276) -> (junction 1271) : {j = j + 1;}
        (junction 1271) -> (junction 1280) [order 2]
        (junction 1272) -> (junction 1274) [order 2]
        (junction 1273) -> (junction 1278) : {StateData(j,2) = 0;
            | m = m+1;}
        (junction 1274) -> (junction 1275) [order 1] : %虽然有发射命令，但是离架计时为0，说明没有发生
            | [info2FSC.ins_FS(j)==1 && info_FSC.count_sprt_msl(j)<=0]
        (junction 1274) -> (junction 1276) [order 2]
        (junction 1275) -> (junction 1277) : {StateData(j,3) = 0;
            | n = n+1;}
        (junction 1277) -> (junction 1276)
        (junction 1278) -> (junction 1277)
        (junction 1279) -> (junction 1278)
        (junction 1280) -> (junction 1281) [order 1] : [Actions.PwrOn||Actions.PwrOff||Actions.FS]
        (junction 1280) -> (junction 1282) [order 2]
        (junction 1281) -> (junction 1283) : {StateInf = 0;}
        (junction 1283) -> (junction 1282)
        (junction 1282) -> (junction 1284)
        (junction 1284) -> (junction 1285) [order 1] : [sum(info2FSC.ins_pwr_on)>0&&m == sum(info2FSC.ins_pwr_on)] % 说明本次没有加电成功的DD
        (junction 1284) -> (junction 1286) [order 2]
        (junction 1285) -> (junction 1287) : {StateInf = 712;}
        (junction 1287) -> (junction 1286)
        (junction 1286) -> (junction 1288)
        (junction 1288) -> (junction 1289) [order 1] : [sum(info2FSC.ins_FS)>0&&n == sum(info2FSC.ins_FS)] % 说明本次没有发射成功的DD
        (junction 1288) -> (junction 1290) [order 2]
        (junction 1289) -> (junction 1291) : {StateInf = 110;}
        (junction 1291) -> (junction 1290)
        (junction 1290) -> (junction 1303) : {StateData0.StateData = StateData;
            | StateData0.StateInf = StateInf;
            | j = 1;}
        (junction 1292) -> (junction 1293) [order 1] : [avl_FS_tgt(j) == 1]
        (junction 1293) -> (junction 1294) [order 1] : % 选了j个目标的第1颗dd
            | [Inds.TgtPwrInd(j,1)]
        (junction 1303) -> (junction 1292) [order 1] : [j<8]
        (junction 1292) -> (junction 1317) [order 2]
        (junction 1293) -> (junction 1295) [order 2] : {DD1 = 0;
            | DD10 = 0; }
        (junction 1294) -> (junction 1296) : %j个目标的第一颗dd编号
            | {DD1 = TargetData(j,5);}
        (junction 1296) -> (junction 1295)
        (junction 1295) -> (junction 1297)
        (junction 1297) -> (junction 1298) [order 1] : [DD1>0]
        (junction 1298) -> (junction 1299) [order 1] : %这颗dd的状态为0
            | [info_FSC.stt_pwr_msl(DD1)==0]
        (junction 1297) -> (junction 1300) [order 2]
        (junction 1298) -> (junction 1301) [order 2] : {DD10 = 1;}
        (junction 1299) -> (junction 1302) : %选中了dd1且dd1状态为0
            | {DD10 = 0;}
        (junction 1301) -> (junction 1300)
        (junction 1302) -> (junction 1301)
        (junction 1300) -> (junction 1304)
        (junction 1317) -> (junction 1303) : {j = j+1;}
        (junction 1303) -> (junction 1316) [order 2]
        (junction 1304) -> (junction 1305) [order 1] : [Inds.TgtPwrInd(j,2)]
        (junction 1304) -> (junction 1306) [order 2] : {DD2 = 0;
            | DD20= 0;}
        (junction 1305) -> (junction 1307) : {DD2 = TargetData(j,6);}
        (junction 1307) -> (junction 1306)
        (junction 1306) -> (junction 1308)
        (junction 1308) -> (junction 1309) [order 1] : [DD2>0]
        (junction 1309) -> (junction 1310) [order 1] : [info_FSC.stt_pwr_msl(DD2)==0]
        (junction 1308) -> (junction 1311) [order 2]
        (junction 1309) -> (junction 1312) [order 2] : {DD20 = 1;}
        (junction 1310) -> (junction 1313) : {DD20 = 0;}
        (junction 1312) -> (junction 1311)
        (junction 1313) -> (junction 1312)
        (junction 1311) -> (junction 1314)
        (junction 1314) -> (junction 1315) [order 1] : % 两颗dd均被选，但是两颗dd的状态均为0
            | % 或者一颗dd选中了，其状态为0，而另一颗dd未选
            | [DD10==0&&DD20==0]
        (junction 1314) -> (junction 1318) [order 2]
        (junction 1315) -> (junction 1319) : {avl_FS_tgt(j) = 0;}
        (junction 1318) -> (junction 1317)
        (junction 1319) -> (junction 1318)
      state PwrOff [parallel]
        settings: executionOrder=2
        (default) -> (junction 1234)
        On.DataProcess1.PwrOff -> (junction 1234)
        (junction 1234) -> (junction 1235) [order 1] : [Actions.PwrOff]
        (junction 1234) -> (junction 1236) [order 2]
        (junction 1235) -> (junction 1237) : {info2FSC.ins_pwr_on = [false;false;false;false;false;false;false;false];
            | info2FSC.ins_pwr_of = [false;false;false;false;false;false;false;false];
            | info2FSC.ins_FS = [false;false;false;false;false;false;false;false];}
        (junction 1237) -> (junction 1236)
        (junction 1236) -> (junction 1240) : {i = 1;}
        (junction 1238) -> (junction 1239) [order 1] : [Inds.TgtPwrInd(i,1)]
        (junction 1240) -> (junction 1238) [order 1] : [i  < 8]
        (junction 1238) -> (junction 1241) [order 2]
        (junction 1239) -> (junction 1242) : {ddInd1 = TargetData(i,5);
            | info2FSC.ins_pwr_of(ddInd1) = true;}
        (junction 1242) -> (junction 1241)
        (junction 1246) -> (junction 1240) : {i = i + 1;}
        (junction 1240) -> (junction 1245) [order 2]
        (junction 1241) -> (junction 1243)
        (junction 1243) -> (junction 1244) [order 1] : [Inds.TgtPwrInd(i,2)]
        (junction 1243) -> (junction 1246) [order 2]
        (junction 1244) -> (junction 1247) : {ddInd1 = TargetData(i,6);
            | info2FSC.ins_pwr_of(ddInd1) = true;}
        (junction 1247) -> (junction 1246)
      state PwrOn [parallel]
        settings: executionOrder=1
        (default) -> (junction 1424)
        On.DataProcess1.PwrOn -> (junction 1424)
        (junction 1424) -> (junction 1425) [order 1] : [Actions.PwrOn]
        (junction 1424) -> (junction 1426) [order 2]
        (junction 1425) -> (junction 1427) : {info2FSC.ins_pwr_on = [false;false;false;false;false;false;false;false];
            | info2FSC.ins_pwr_of = [false;false;false;false;false;false;false;false];
            | info2FSC.ins_FS = [false;false;false;false;false;false;false;false];}
        (junction 1427) -> (junction 1426)
        (junction 1428) -> (junction 1429) [order 1] : [Inds.TgtPwrInd(i,1)]
        (junction 1432) -> (junction 1428) [order 1] : [i  < 8]
        (junction 1426) -> (junction 1432) : {i = 1;}
        (junction 1428) -> (junction 1430) [order 2]
        (junction 1429) -> (junction 1431) : {ddInd1 = TargetData(i,5);
            | info2FSC.ins_pwr_on(ddInd1) = true;}
        (junction 1431) -> (junction 1430)
        (junction 1430) -> (junction 1433)
        (junction 1435) -> (junction 1432) : {i = i + 1;}
        (junction 1432) -> (junction 1437) [order 2]
        (junction 1433) -> (junction 1434) [order 1] : [Inds.TgtPwrInd(i,2)]
        (junction 1433) -> (junction 1435) [order 2]
        (junction 1434) -> (junction 1436) : {ddInd1 = TargetData(i,6);
            | info2FSC.ins_pwr_on(ddInd1) = true;}
        (junction 1436) -> (junction 1435)
      state Out1 = init_info2FSC [function]
  (default) -> Init
  Init -> On : after(1,sec)
  data: Out1 function_output double size=�; Out1 function_output Bus: BusObject_info_CC2FSC; TargetDataLD input Bus: TgtDataLDBusObject size=1; Inds input Bus: ChooseBusObject size=1; TargetData output double size=[8 7]; VtgtData output size=[8 3]; avl_asn_tgt output double size=8; avl_asn_msl output double size=8; avl_pwr_tgt output double size=8; avl_FS_tgt output double size=8; StateData0 output Bus: StateBusObject; i local; ddInd local; info2FSC output Bus: BusObject_info_CC2FSC size=1; ddInd1 local; Actions input Bus: ActionBusObject size=1; info_FSC input Bus: BusObject_info_FSC2CC size=1; StateData local double size=[8 3]; StateInf local double size=1; m local; n local; j local; DD1 local; DD2 local; Para_FS0 local Bus: BusObject_msg_FSC2msl; DD10 local; DD20 local; struct_info_CC2FSC parameter
